simulink model "model4tuningPIDs"  (R2018b)
settings: Solver=VariableStepAuto  StartTime=0.0  StopTime=10.0  RelTol=1e-3
values from neighbouring files (symbols this model uses):
  Lf = 2.56    [makeBikeModel.m]    (also in makePlants.m; tunePIDs.m = 0.55)
  Lr = 1.02    [makeBikeModel.m]    (also in makePlants.m; tunePIDs.m = 0.525)
undefined symbols (not defined in the file or in its folder): plants
libraries: simulink x1
settings Model: Creator=lachc  LastModifiedBy=lachc

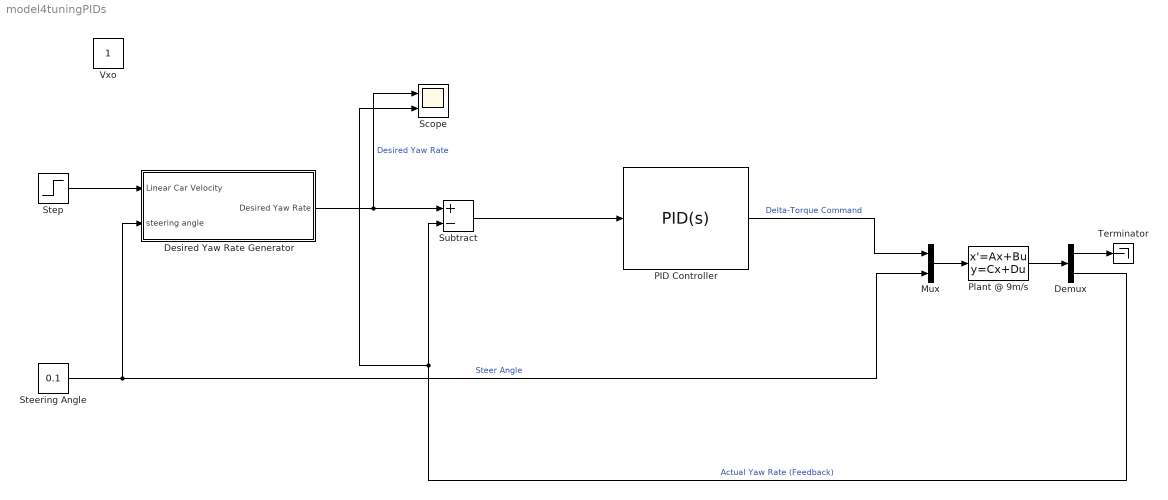
== system model4tuningPIDs ==
  Demux : Demux  Outputs=2
  Desired Yaw Rate Generator : Subsystem
  Mux : Mux  Inputs=2
  PID Controller : simulink/Continuous/PID Controller  Controller=PID  Form=Parallel  TimeDomain=Continuous-time  SampleTime=-1  IntegratorMethod=Forward Euler  FilterMethod=Forward Euler  ControllerParametersSource=internal  P=201.998725149977  I=53139.3625453069  D=0  UseFilter=on  N=100  TunerSelectOption=Transfer Function Based (PID Tuner App)  InitialConditionSource=internal  InitialConditionForIntegrator=0  InitialConditionForFilter=0  DifferentiatorICPrevScaledInput=0  ExternalReset=none  TrackingMode=off  Kt=1  LimitOutput=on  UpperSaturationLimit=180  LowerSaturationLimit=0  LinearizeAsGain=off  AntiWindupMode=clamping  Kb=1  POutMin=[]  POutMax=[]  IOutMin=[]  IOutMax=[]  DOutMin=[]  DOutMax=[]  NOutMin=[]  NOutMax=[]  SumOutMin=[]  SumOutMax=[]  SaturationOutMin=[]  SaturationOutMax=[]  PParamMin=[]  PParamMax=[]  IParamMin=[]  IParamMax=[]  DParamMin=[]  DParamMax=[]  NParamMin=[]  NParamMax=[]  KbParamMin=[]  KbParamMax=[]  KtParamMin=[]  KtParamMax=[]  KbOutMin=[]  KbOutMax=[]  KtOutMin=[]  KtOutMax=[]  IntegratorOutMin=[]  IntegratorOutMax=[]  FilterOutMin=[]  FilterOutMax=[]  SumI1OutMin=[]  SumI1OutMax=[]  SumI2OutMin=[]  SumI2OutMax=[]  SumI3OutMin=[]  SumI3OutMax=[]  SumI4OutMin=[]  SumI4OutMax=[]  SumDOutMin=[]  SumDOutMax=[]  DifferentiatorOutMin=[]  DifferentiatorOutMax=[]  FilterDiffOutCoefMin=[]  FilterDiffOutCoefMax=[]  ReciprocalOutMin=[]  ReciprocalOutMax=[]  SumDenOutMin=[]  SumDenOutMax=[]  SumNumOutMin=[]  SumNumOutMax=[]  DivideOutMin=[]  DivideOutMax=[]  IntegratorContinuousStateAttributes=''  IntegratorStateMustResolveToSignalObject=off  IntegratorRTWStateStorageClass=Auto  FilterContinuousStateAttributes=''  FilterStateMustResolveToSignalObject=off  FilterRTWStateStorageClass=Auto  ParallelPVariant=InternalParameters  IdealPVariant=Disabled  IVariant=InternalParameters  DVariant=InternalParameters  IntegratorVariant=Continuous  SatVariant=Enabled  AWVariant=ContClampingParallel  PCopyVariant=Disabled  TRVariant=Disabled  FdbkBlocksVariant=Forward  IdealPFdbkVariant=Disabled  SatFdbkVariant=Disabled  DerivativeFilterVariant=ContFilter  NVariant=InternalParameters  NCopyVariant=Disabled  FilterICVariant=InternalICsFilter  IntegratorICVariant=InternalICs  ExternalResetVariant=Disabled  TRSumVariant=Passthrough  SumFdbkVariant=Disabled  SumVariant=Sum_PID
  Plant @ 9m/s : StateSpace  A=plants(:,:,1).A  B=plants(:,:,1).B  C=plants(:,:,1).C  D=plants(:,:,1).D  InitialCondition=0  ContinuousStateAttributes={'V_lat','yaw_rate'}
  Scope : Scope  NumInputPorts=2
  Steering Angle : Constant  Value=0.1
  Step : Step  SampleTime=0
  Subtract : Sum  Inputs=+-
  Terminator : Terminator
  Vxo : Constant
  wires:
  Demux/1 -> Terminator/1
  Steering Angle/1 -> Desired Yaw Rate Generator/2(steering angle), Mux/2  "Steer Angle"
  PID Controller/1 -> Mux/1  "Delta-Torque Command"
  Subtract/1 -> PID Controller/1
  Demux/2 -> Scope/2, Subtract/2  "Actual Yaw Rate (Feedback)"
  Desired Yaw Rate Generator/1(Desired Yaw Rate) -> Scope/1, Subtract/1  "Desired Yaw Rate"
  Step/1 -> Desired Yaw Rate Generator/1(Linear Car Velocity)
  Mux/1 -> Plant @ 9m/s/1
  Plant @ 9m/s/1 -> Demux/1

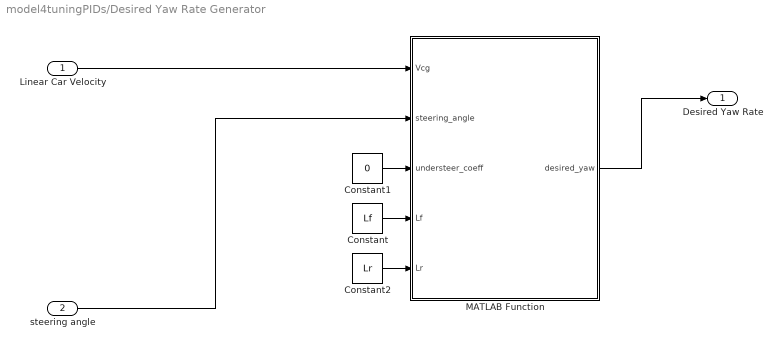
== system model4tuningPIDs/Desired Yaw Rate Generator ==
  Linear Car Velocity : Inport
  steering angle : Inport  Port=2
  Constant : Constant  Value=Lf
  Constant1 : Constant  Value=0
  Constant2 : Constant  Value=Lr
  MATLAB Function : MATLAB Function  TreatAsAtomicUnit=on
  Desired Yaw Rate : Outport
  wires:
  Constant1/1 -> MATLAB Function/3(understeer_coeff)
  steering angle/1 -> MATLAB Function/2(steering_angle)
  MATLAB Function/1(desired_yaw) -> Desired Yaw Rate/1
  Linear Car Velocity/1 -> MATLAB Function/1(Vcg)
  Constant2/1 -> MATLAB Function/5(Lr)
  Constant/1 -> MATLAB Function/4(Lf)

== matlab function model4tuningPIDs/Desired Yaw Rate Generator/MATLAB Function ==
  data: Vcg input; desired_yaw output; steering_angle input; understeer_coeff input; Lf input; Lr input
function desired_yaw = desiredYaw(Vcg , steering_angle, understeer_coeff, Lf, Lr)
desired_yaw = 0;
desired_yaw = Vcg*steering_angle/((Lf*Lr) + understeer_coeff*Vcg^2);
